simulink model "nonlinearQuad"  (R2015b)
settings: Solver=VariableStepAuto  StartTime=0.0  StopTime=10.0  RelTol=1e-3
model workspace (MAT data in the model file):
  op_trim1 : opcond.OperatingReport (value not decoded)
values from neighbouring files (symbols this model uses):
  K = lqr(sysd,Q,R)    [ControllerDesign.m]    (also in feedback_gain.m = [79.0556825830553 2.2360679774993049 -1.5811388299925784 -1.)
settings Model: Creator=marcus  LastModifiedBy=marcus
settings DataIOCC: ExternalInput=getinputstruct(op_trim1)  InitialState=getstatestruct(op_trim1)  SaveFormat=Structure

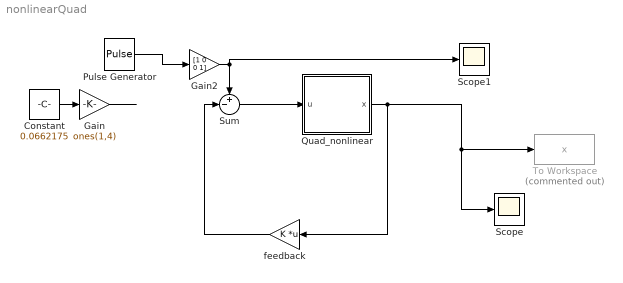
== system nonlinearQuad ==
  Constant : Constant  Value=0.0662175
  Gain : Gain  Gain=ones(1,4)
  Gain2 : Gain  Gain=[1 0 0 1]
  Pulse Generator : DiscretePulseGenerator  PulseType=Time based  Period=10  PhaseDelay=1
  Quad_nonlinear : Subsystem
  Scope : Scope
  Scope1 : Scope
  Sum : Sum  Inputs=+-|
  To Workspace : ToWorkspace  Commented=on  VariableName=x  SaveFormat=Timeseries  SampleTime=-1
  feedback : Gain  Gain=K  Multiplication=Matrix(K*u)
  wires:
  Constant/1 -> Gain/1
  Quad_nonlinear/1(x) -> feedback/1, To Workspace/1, Scope/1
  Gain/1 -> ?
  feedback/1 -> Sum/2
  Pulse Generator/1 -> Gain2/1
  Gain2/1 -> Sum/1, Scope1/1
  Sum/1 -> Quad_nonlinear/1(u)

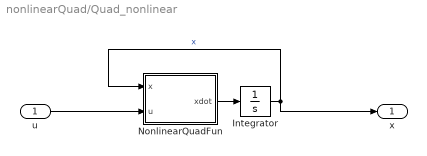
== system nonlinearQuad/Quad_nonlinear ==
  u : Inport
  Integrator : Integrator  InitialCondition=zeros(12,1)
  NonlinearQuadFun : MATLAB Function  TreatAsAtomicUnit=on
  x : Outport
  wires:
  u/1 -> NonlinearQuadFun/2(u)
  NonlinearQuadFun/1(xdot) -> Integrator/1
  Integrator/1 -> x/1, NonlinearQuadFun/1(x)  "x"

== matlab function nonlinearQuad/Quad_nonlinear/NonlinearQuadFun ==
  data: x input; u input; xdot output
function xdot = fcn(x,u)
%#codegen

% extract states and inputs
v=x(4:6);

r=x(7);
p=x(8);
y=x(9);

w1=x(10);
w2=x(11);
w3=x(12);

T=sum(u);
T1=u(1);
T2=u(2);
T3=u(3);
T4=u(4);

%constants
g=9.81;
m=0.027;
b=1e-3;
k=b;
d=0.1;
Ix = 1.395e-5;
Iy = 1.436e-5;
Iz = 2.173e-5;

invJ=inv([Ix,0,0;
            0,Iy,0;
            0,0,Iz]);
        
invBigT=inv([1,0,-sin(p);
            0,cos(r),sin(r)*cos(p);
            0,-sin(r),cos(p)*cos(r)]);

As=[0 -d 0 d;
    d 0 -d 0;
    k/b -k/b k/b -k/b];

R=[cos(r)*cos(y)-cos(p)*sin(r)*sin(y), -cos(y)*sin(r)-cos(r)*cos(p)*sin(y), sin(p)*sin(y);
     cos(p)*cos(y)*sin(r)+cos(r)*sin(y), cos(r)*cos(p)*cos(y)-sin(r)*sin(y), -cos(y)*sin(p);
     sin(r)*sin(p), cos(r)*sin(p), cos(p) ];


%equations
xyzdot=v;

vdot=[0;0;g/m] - R*[0;0;T/m];
    
rpydot=invBigT*[w1;w2;w3];

wdot=invJ*As*[T1;T2;T3;T4] - invJ*[(Iy-Iz)*w2*w3;
                                         (Iz-Ix)*w1*w3;
                                         (Ix-Iy)*w1*w2];


xdot = [xyzdot; vdot; rpydot; wdot];
